simulink model "simulink_traverse_control"  (R2022b)
settings: Solver=ode5  StartTime=0.0  StopTime=sim_time  FixedStep=T  RelTol=1e-3
values from neighbouring files (symbols this model uses):
  T = 1/srate    (= 0.001)    [setup_DAQ_simulink.m]
undefined symbols (not defined in the file or in its folder): freq, heave1, National_Instruments, PCIe
libraries: sldrtlib x12
settings Model: SimulationMode=external  ExtModeTrigDuration=100000  Creator=ehandyca  LastModifiedBy=ehandyca
settings DataIOCC: ReturnWorkspaceOutputs=off
settings HardwareCC: ProdBitPerLong=64  ProdHWDeviceType=Intel->x86-64 (Linux 64)
settings RTWCC: Description=Simulink Desktop Real-Time  SystemTargetFile=sldrt.tlc  TemplateMakefile=sldrt.tmf  RTWCompilerOptimization=on
settings CodeAppCC: MaxIdLength=95
settings SimulinkDesktopRealTimeCC: TargetLibSuffix=_sldrt.a  TargetPreCompLibLocation=C:\Program Files\MATLAB\R2022b\toolbox\sldrt\lib\win64

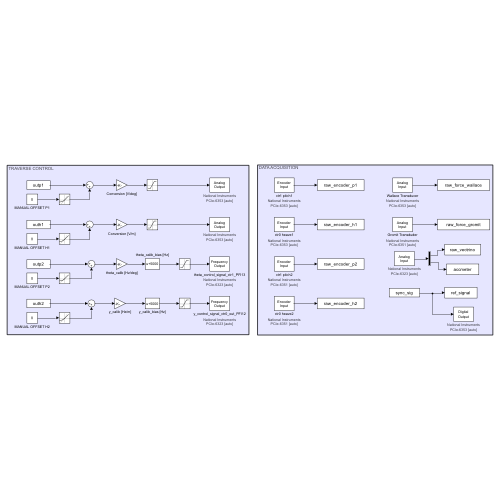
[thumbnail: Simulink's stored preview of the top-level diagram]
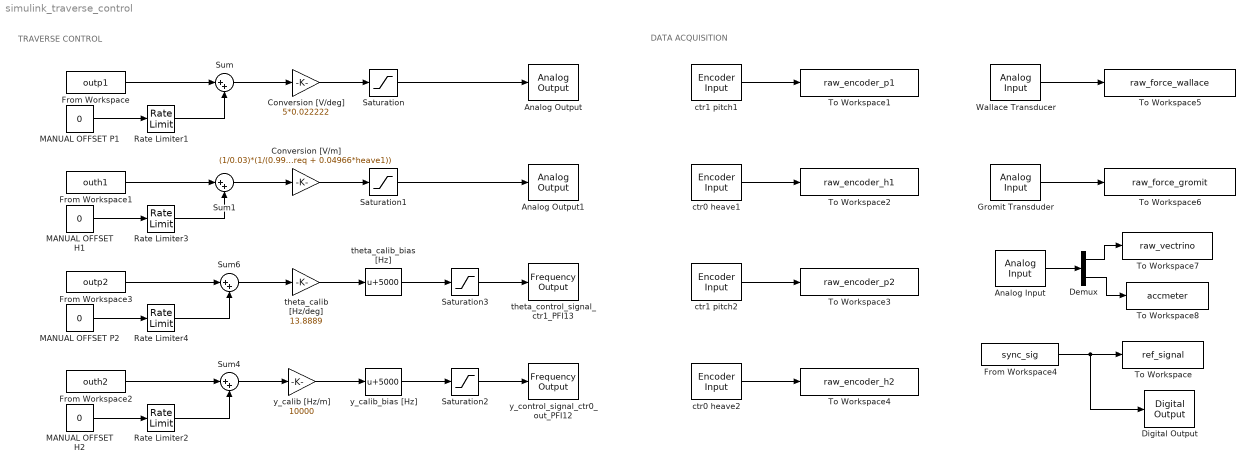
== system simulink_traverse_control ==
  note: TRAVERSE CONTROL
  note: DATA ACQUISITION
  Analog Input : sldrtlib/Analog Input  SampleTime=T  MaxMissedTicks=10  ShowMissedTicks=off  YieldWhenWaiting=off  DrvName=National_Instruments/PCIe-6323  DrvAddress=4294967295  DrvOptions=[0 3 0 3 3 3 3]  Channels=[17,18,19,20,21]  RangeMode=1  VoltRange=1  DataType=1
      settings: AttributesFormatString=National Instruments\nPCIe-6323 [auto]
  Analog Output : sldrtlib/Analog Output  SampleTime=T  MaxMissedTicks=10  ShowMissedTicks=off  YieldWhenWaiting=off  DrvName=National_Instruments/PCIe-6353  DrvAddress=4294967295  DrvOptions=[1 57440 0 2 2 2 2]  Channels=[3]  RangeMode=1  VoltRange=1  InitialValue=[]  FinalValue=[]
      settings: AttributesFormatString=National Instruments\nPCIe-6353 [auto]
  Analog Output1 : sldrtlib/Analog Output  SampleTime=T  MaxMissedTicks=10  ShowMissedTicks=off  YieldWhenWaiting=off  DrvName=National_Instruments/PCIe-6353  DrvAddress=4294967295  DrvOptions=[1 57440 0 2 2 2 2]  Channels=[4]  RangeMode=1  VoltRange=1  InitialValue=[]  FinalValue=[]
      settings: AttributesFormatString=National Instruments\nPCIe-6353 [auto]
  Conversion [V/deg] : Gain  Gain=5*0.022222
  Conversion [V/m] : Gain  Gain=(1/0.03)*(1/(0.991-0.01095*freq + 0.04966*heave1))
  Demux : Demux  Outputs=[4, 1]
  Digital Output : sldrtlib/Digital Output  SampleTime=T  MaxMissedTicks=10  ShowMissedTicks=off  YieldWhenWaiting=off  DrvName=National_Instruments/PCIe-6353  DrvAddress=4294967295  DrvOptions=[1 57440 0 2 2 2 2]  Channels=[15]  BitMode=1  InitialValue=[]  FinalValue=[]
      settings: AttributesFormatString=National Instruments\nPCIe-6353 [auto]
  From Workspace : FromWorkspace  VariableName=outp1  SampleTime=T  Interpolate=off  OutputAfterFinalValue=Holding final value
  From Workspace1 : FromWorkspace  VariableName=outh1  SampleTime=T  Interpolate=off  OutputAfterFinalValue=Holding final value
  From Workspace2 : FromWorkspace  VariableName=outh2  SampleTime=T  Interpolate=off  OutputAfterFinalValue=Holding final value
  From Workspace3 : FromWorkspace  VariableName=outp2  SampleTime=T  Interpolate=off  OutputAfterFinalValue=Holding final value
  From Workspace4 : FromWorkspace  VariableName=sync_sig  SampleTime=T  OutputAfterFinalValue=Holding final value
  Gromit Transduder : sldrtlib/Analog Input  SampleTime=T  MaxMissedTicks=10  ShowMissedTicks=off  YieldWhenWaiting=off  DrvName=National_Instruments/PCIe-6351  DrvAddress=4294967295  DrvOptions=[1 0 0 2 2 2 2]  Channels=[1:6]  RangeMode=1  VoltRange=1  DataType=1
      settings: AttributesFormatString=National Instruments\nPCIe-6351 [auto]
  MANUAL OFFSET H1 : Constant  Value=0
  MANUAL OFFSET H2 : Constant  Value=0
  MANUAL OFFSET P1 : Constant  Value=0
  MANUAL OFFSET P2 : Constant  Value=0
  Rate Limiter1 : RateLimiter  RisingSlewLimit=15  FallingSlewLimit=-15  SampleTimeMode=inherited
  Rate Limiter2 : RateLimiter  RisingSlewLimit=0.05  FallingSlewLimit=-0.05  SampleTimeMode=inherited
  Rate Limiter3 : RateLimiter  RisingSlewLimit=0.05  FallingSlewLimit=-0.05  SampleTimeMode=inherited
  Rate Limiter4 : RateLimiter  RisingSlewLimit=15  FallingSlewLimit=-15  SampleTimeMode=inherited
  Saturation : Saturate  UpperLimit=10  LowerLimit=-10
  Saturation1 : Saturate  UpperLimit=10  LowerLimit=-10
  Saturation2 : Saturate  UpperLimit=10000  LowerLimit=5000
  Saturation3 : Saturate  UpperLimit=9200  LowerLimit=5000
  Sum{,1,4,6} (4 alike) : Sum  Inputs=|++
  To Workspace : ToWorkspace  VariableName=ref_signal  SampleTime=T
      settings: Save2DSignal=2-D array (concatenate along first dimension)
  To Workspace1 : ToWorkspace  VariableName=raw_encoder_p1  SampleTime=T
      settings: Save2DSignal=2-D array (concatenate along first dimension)
  To Workspace2 : ToWorkspace  VariableName=raw_encoder_h1  SampleTime=T
      settings: Save2DSignal=2-D array (concatenate along first dimension)
  To Workspace3 : ToWorkspace  VariableName=raw_encoder_p2  SampleTime=T
      settings: Save2DSignal=2-D array (concatenate along first dimension)
  To Workspace4 : ToWorkspace  VariableName=raw_encoder_h2  SampleTime=T
      settings: Save2DSignal=2-D array (concatenate along first dimension)
  To Workspace5 : ToWorkspace  VariableName=raw_force_wallace  SampleTime=T
      settings: Save2DSignal=2-D array (concatenate along first dimension)
  To Workspace6 : ToWorkspace  VariableName=raw_force_gromit  SampleTime=T
      settings: Save2DSignal=2-D array (concatenate along first dimension)
  To Workspace7 : ToWorkspace  VariableName=raw_vectrino  SampleTime=T
      settings: Save2DSignal=2-D array (concatenate along first dimension)
  To Workspace8 : ToWorkspace  VariableName=accmeter  SampleTime=T
      settings: Save2DSignal=2-D array (concatenate along first dimension)
  Wallace Transducer : sldrtlib/Analog Input  SampleTime=T  MaxMissedTicks=10  ShowMissedTicks=off  YieldWhenWaiting=off  DrvName=National_Instruments/PCIe-6353  DrvAddress=4294967295  DrvOptions=[1 57440 0 2 2 2 2]  Channels=[1,2,3,4,5,6]  RangeMode=1  VoltRange=1  DataType=1
      settings: AttributesFormatString=National Instruments\nPCIe-6353 [auto]
  ctr0 heave1 : sldrtlib/Encoder Input  SampleTime=T  MaxMissedTicks=10  ShowMissedTicks=off  YieldWhenWaiting=off  DrvName=National_Instruments/PCIe-6353  DrvAddress=4294967295  DrvOptions=[1 57440 0 2 2 2 2]  Channels=1  QuadMode=3  IndexPulse=1  InputFilter=Inf  DataType=1
      settings: AttributesFormatString=National Instruments\nPCIe-6353 [auto]
  ctr0 heave2 : sldrtlib/Encoder Input  SampleTime=T  MaxMissedTicks=10  ShowMissedTicks=off  YieldWhenWaiting=off  DrvName=National_Instruments/PCIe-6351  DrvAddress=4294967295  DrvOptions=[1 0 0 2 2 2 2]  Channels=1  QuadMode=3  IndexPulse=2  InputFilter=Inf  DataType=1
      settings: AttributesFormatString=National Instruments\nPCIe-6351 [auto]
  ctr1 pitch1 : sldrtlib/Encoder Input  SampleTime=T  MaxMissedTicks=10  ShowMissedTicks=off  YieldWhenWaiting=off  DrvName=National_Instruments/PCIe-6353  DrvAddress=4294967295  DrvOptions=[1 57440 0 2 2 2 2]  Channels=2  QuadMode=3  IndexPulse=1  InputFilter=Inf  DataType=1
      settings: AttributesFormatString=National Instruments\nPCIe-6353 [auto]
  ctr1 pitch2 : sldrtlib/Encoder Input  SampleTime=T  MaxMissedTicks=10  ShowMissedTicks=off  YieldWhenWaiting=off  DrvName=National_Instruments/PCIe-6351  DrvAddress=4294967295  DrvOptions=[1 0 0 2 2 2 2]  Channels=2  QuadMode=3  IndexPulse=2  InputFilter=Inf  DataType=1
      settings: AttributesFormatString=National Instruments\nPCIe-6351 [auto]
  theta_calib [Hz/deg] : Gain  Gain=13.8889
  theta_calib_bias [Hz] : Bias  Bias=5000  SaturateOnIntegerOverflow=off
  theta_control_signal_ctr1_PFI13 : sldrtlib/Frequency Output  SampleTime=T  MaxMissedTicks=10  ShowMissedTicks=off  YieldWhenWaiting=off  DrvName=National_Instruments/PCIe-6323  DrvAddress=4294967295  DrvOptions=[0 3 0 3 3 3 3]  Channels=2  FrequencySource=2  Frequency=[]  FrequencyFinalValue=[]  DutySource=1  Duty=0.5  DutyFinalValue=[]
      settings: AttributesFormatString=National Instruments\nPCIe-6323 [auto]
  y_calib [Hz/m] : Gain  Gain=10000
  y_calib_bias [Hz] : Bias  Bias=5000  SaturateOnIntegerOverflow=off
  y_control_signal_ctr0_out_PFI12 : sldrtlib/Frequency Output  SampleTime=T  MaxMissedTicks=10  ShowMissedTicks=off  YieldWhenWaiting=off  DrvName=National_Instruments/PCIe-6323  DrvAddress=4294967295  DrvOptions=[0 3 0 3 3 3 3]  Channels=1  FrequencySource=2  Frequency=[]  FrequencyFinalValue=[]  DutySource=1  Duty=0.5  DutyFinalValue=[]
      settings: AttributesFormatString=National Instruments\nPCIe-6323 [auto]
  wires:
  Conversion [V/deg]/1 -> Saturation/1
  Sum/1 -> Conversion [V/deg]/1
  Sum1/1 -> Conversion [V/m]/1
  Conversion [V/m]/1 -> Saturation1/1
  Saturation1/1 -> Analog Output1/1
  Saturation/1 -> Analog Output/1
  y_calib_bias [Hz]/1 -> Saturation2/1
  Saturation2/1 -> y_control_signal_ctr0_out_PFI12/1
  Sum4/1 -> y_calib [Hz/m]/1
  y_calib [Hz/m]/1 -> y_calib_bias [Hz]/1
  theta_calib [Hz/deg]/1 -> theta_calib_bias [Hz]/1
  Sum6/1 -> theta_calib [Hz/deg]/1
  theta_calib_bias [Hz]/1 -> Saturation3/1
  Saturation3/1 -> theta_control_signal_ctr1_PFI13/1
  ctr0 heave1/1 -> To Workspace2/1
  ctr1 pitch1/1 -> To Workspace1/1
  ctr0 heave2/1 -> To Workspace4/1
  ctr1 pitch2/1 -> To Workspace3/1
  Wallace Transducer/1 -> To Workspace5/1
  Rate Limiter1/1 -> Sum/2
  MANUAL OFFSET P1/1 -> Rate Limiter1/1
  From Workspace/1 -> Sum/1
  Rate Limiter3/1 -> Sum1/2
  MANUAL OFFSET H1/1 -> Rate Limiter3/1
  From Workspace1/1 -> Sum1/1
  From Workspace3/1 -> Sum6/1
  MANUAL OFFSET P2/1 -> Rate Limiter4/1
  Rate Limiter4/1 -> Sum6/2
  MANUAL OFFSET H2/1 -> Rate Limiter2/1
  Rate Limiter2/1 -> Sum4/2
  From Workspace2/1 -> Sum4/1
  Gromit Transduder/1 -> To Workspace6/1
  Analog Input/1 -> Demux/1
  Demux/2 -> To Workspace8/1
  Demux/1 -> To Workspace7/1
  From Workspace4/1 -> Digital Output/1, To Workspace/1
